simulink model "sineCosine"  (R2024b)
settings: Solver=VariableStepAuto  StartTime=0.0  StopTime=20.0  RelTol=1e-3
libraries: simulink x2, SignalEditorBlockLib x1
settings Model: Creator=optimus  LastModifiedBy=optimus

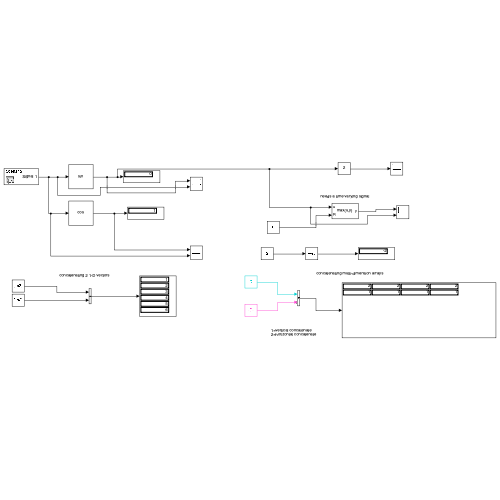
[thumbnail: Simulink's stored preview of the top-level diagram]
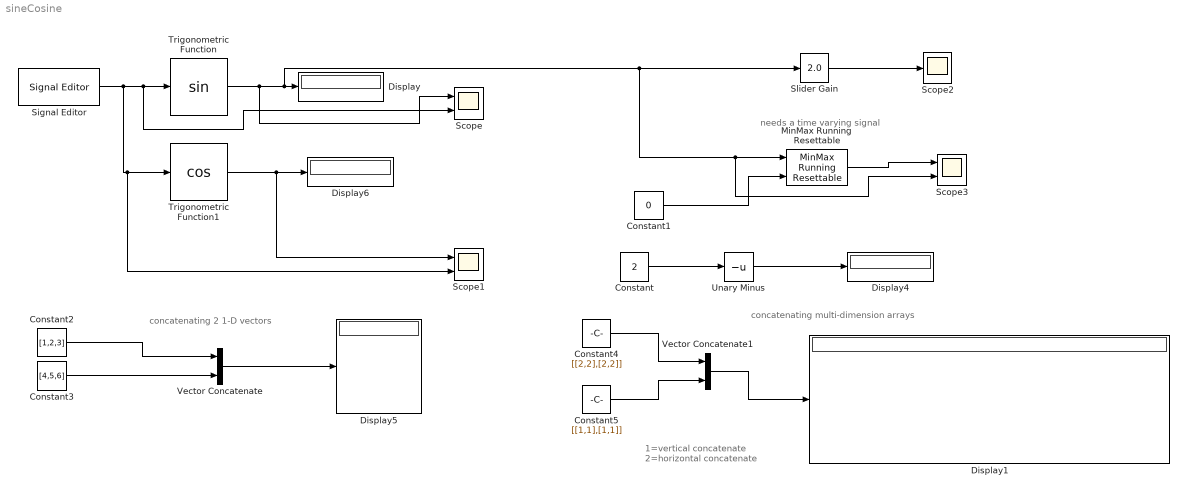
== system sineCosine ==
  note: 1=vertical concatenate
      | 2=horizontal concatenate
  note: concatenating multi-dimension arrays
  note: concatenating 2 1-D vectors
  note: needs a time varying signal
  Constant : Constant  Value=2
  Constant1 : Constant  Value=0
  Constant2 : Constant  Value=[1,2,3]
  Constant3 : Constant  Value=[4,5,6]
  Constant4 : Constant  Value=[[2,2],[2,2]]  VectorParams1D=off
  Constant5 : Constant  Value=[[1,1],[1,1]]  VectorParams1D=off
  Display{,1,4..6} (5 alike) : Display
  MinMax Running Resettable : simulink/Math Operations/MinMax Running Resettable  Function=max  vinit=0.0
  Scope : Scope  NumInputPorts=2
  Scope1 : Scope  NumInputPorts=2
  Scope2 : Scope
  Scope3 : Scope  NumInputPorts=2
  Signal Editor : SignalEditorBlockLib/Signal Editor  FileName=/Users/optimus/Documents/Matlab_Simulink_Projects/mathOperations/signal_step.mat  ActiveScenario=Scenario  ActiveSignal=Signal 1  IsBus=off  OutputBusObjectStr=Bus: BusObject  SampleTime=0  Interpolate=off  ZeroCross=off  OutputAfterFinalValue=Setting to zero  Unit=inherit  PreserveSignalName=on  ApplySigPropsToAllScenarios=on  ApplySigPropsToAllSignals=off
  Slider Gain : simulink/Math Operations/Slider Gain  gain=2.0  low=0  high=2
  Trigonometric Function : Trigonometry
  Trigonometric Function1 : Trigonometry  Operator=cos
  Unary Minus : UnaryMinus
  Vector Concatenate : Concatenate
  Vector Concatenate1 : Concatenate  Mode=Multidimensional array
  wires:
  Slider Gain/1 -> Scope2/1
  MinMax Running Resettable/1 -> Scope3/1
  Unary Minus/1 -> Display4/1
  Vector Concatenate/1 -> Display5/1
  Trigonometric Function1/1 -> Scope1/1, Display6/1
  Signal Editor/1 -> Scope1/2, Trigonometric Function1/1, Scope/2, Trigonometric Function/1
  Trigonometric Function/1 -> Scope/1, Scope3/2, MinMax Running Resettable/1, Slider Gain/1, Display/1
  Constant1/1 -> MinMax Running Resettable/2
  Constant/1 -> Unary Minus/1
  Constant3/1 -> Vector Concatenate/2
  Constant2/1 -> Vector Concatenate/1
  Vector Concatenate1/1 -> Display1/1
  Constant5/1 -> Vector Concatenate1/2
  Constant4/1 -> Vector Concatenate1/1
